simulink model "realInductor"  (R2013a)
settings: Solver=ode45  StartTime=0.0  StopTime=10.0  RelTol=1e-3
values from neighbouring files (symbols this model uses):
  JR = 7.3E-9    [dataDict_galvoLSK040EF.sldd]    (also in dataDict_galvoMod6860.sldd = 6.0E-8
  L = 0.0018    [dataDict_galvoLSK040EF.sldd]    (also in dataDict_galvoMod6860.sldd = 0.00016
  RL = 2.3    [dataDict_galvoLSK040EF.sldd]    (also in dataDict_galvoMod6860.sldd = 1.5
undefined symbols (not defined in the file or in its folder): BF, KME
settings Model: Creator=mainster  LastModifiedBy=mainster

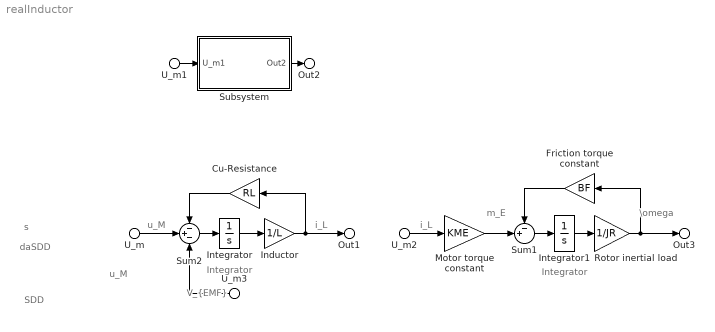
== system realInductor ==
  note: SDD
  note: daSDD
  note: s
  note: u_M
  note: Integrator
  note: Integrator
  note: u_M
  note: i_L
  note: m_E
  note: \omega
  note: i_L
  note: V_{EMF}
  U_m : Inport
  U_m2 : Inport  Port=2
  U_m1 : Inport  Port=3
  U_m3 : Inport  Port=4
  Cu-Resistance : Gain  Gain=RL
  Friction torque constant : Gain  Gain=BF
  Inductor : Gain  Gain=1/L
  Integrator : Integrator
  Integrator1 : Integrator
  Motor torque constant : Gain  Gain=KME
  Rotor inertial load : Gain  Gain=1/JR
  Subsystem : Subsystem
  Sum1 : Sum  Inputs=-+|
  Sum2 : Sum  Inputs=-+-
  Out1 : Outport
  Out3 : Outport  Port=2
  Out2 : Outport  Port=3
  wires:
  Sum2/1 -> Integrator/1
  Integrator/1 -> Inductor/1
  Inductor/1 -> Out1/1, Cu-Resistance/1
  Cu-Resistance/1 -> Sum2/1
  U_m2/1 -> Motor torque constant/1
  Rotor inertial load/1 -> Out3/1, Friction torque constant/1
  Friction torque constant/1 -> Sum1/1
  Integrator1/1 -> Rotor inertial load/1
  Sum1/1 -> Integrator1/1
  Motor torque constant/1 -> Sum1/2
  U_m1/1 -> Subsystem/1(U_m1)
  Subsystem/1(Out2) -> Out2/1
  U_m/1 -> Sum2/2
  U_m3/1 -> Sum2/3

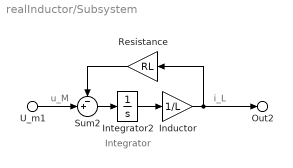
== system realInductor/Subsystem ==
  note: Integrator
  note: u_M
  note: i_L
  U_m1 : Inport
  Inductor : Gain  Gain=1/L
  Integrator2 : Integrator
  Resistance : Gain  Gain=RL
  Sum2 : Sum  Inputs=-+|
  Out2 : Outport
  wires:
  U_m1/1 -> Sum2/2
  Sum2/1 -> Integrator2/1
  Inductor/1 -> Out2/1, Resistance/1
  Integrator2/1 -> Inductor/1
  Resistance/1 -> Sum2/1
